simulink model "OpenLoopBraking"  (R2026b)
undefined symbols (not defined in the file): CtrlBcuTrlrBrkGain
settings Model: Creator=The MathWorks, Inc.  LastModifiedBy=The MathWorks, Inc.

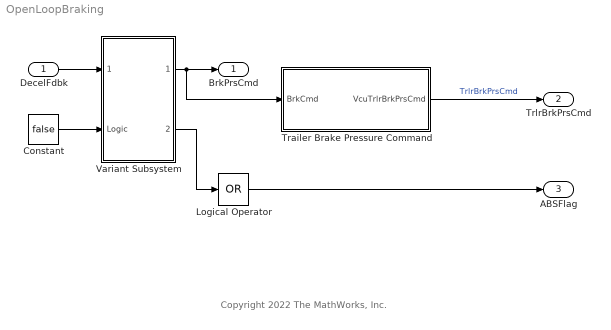
== system OpenLoopBraking ==
  note: Copyright 2022 The MathWorks, Inc.
  DecelFdbk : Inport  OutDataTypeStr=double  PortDimensions=1
  Constant : Constant  Value=false
  Logical Operator : Logic  Operator=OR  Inputs=1  AllPortsSameDT=off  OutDataTypeStr=boolean
  Trailer Brake Pressure Command : Subsystem
  Variant Subsystem : Subsystem  Variant=on  VariantControlMode=label  LabelModeActiveChoice=TwoAxle
  BrkPrsCmd : Outport  OutDataTypeStr=double  VectorParamsAs1DForOutWhenUnconnected=off
  TrlrBrkPrsCmd : Outport  Port=2  PortDimensions=6  VectorParamsAs1DForOutWhenUnconnected=off
  ABSFlag : Outport  Port=3
  wires:
  Variant Subsystem/2(ABSFlag) -> Logical Operator/1
  Constant/1 -> Variant Subsystem/2(Logic)
  Variant Subsystem/1(BrkCmd) -> Trailer Brake Pressure Command/1(BrkCmd), BrkPrsCmd/1
  DecelFdbk/1 -> Variant Subsystem/1(DecelFdbk)
  Trailer Brake Pressure Command/1(VcuTrlrBrkPrsCmd) -> TrlrBrkPrsCmd/1  "TrlrBrkPrsCmd"
  Logical Operator/1 -> ABSFlag/1

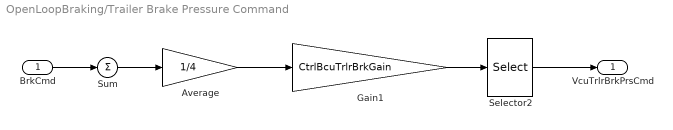
== system OpenLoopBraking/Trailer Brake Pressure Command ==
  BrkCmd : Inport
  Average : Gain  Gain=1/4
  Gain1 : Gain  Gain=CtrlBcuTrlrBrkGain
  Selector2 : Selector  InputPortWidth=1  IndexOptions=Index vector (dialog)  Indices=[1 1 1 1 1 1]  OutputSizes=1  RuntimeRangeChecks=off
  Sum : Sum  Inputs=+
  VcuTrlrBrkPrsCmd : Outport
  wires:
  Gain1/1 -> Selector2/1
  Average/1 -> Gain1/1
  BrkCmd/1 -> Sum/1
  Sum/1 -> Average/1
  Selector2/1 -> VcuTrlrBrkPrsCmd/1

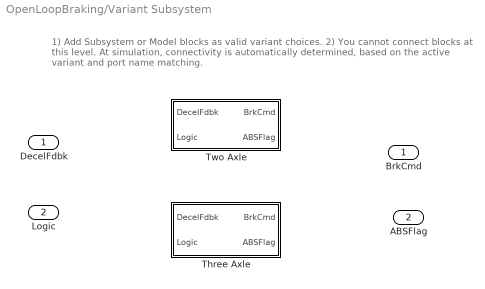
== system OpenLoopBraking/Variant Subsystem ==
  note: 1) Add Subsystem or Model blocks as valid variant choices.
      | 2) You cannot connect blocks at this level. At simulation, connectivity is automatically
      | determined, based on the active variant and port name matching.
  DecelFdbk : Inport
  Logic : Inport  Port=2
  Three Axle : Subsystem  VariantControl=ThreeAxle
  Two Axle : Subsystem  VariantControl=TwoAxle
  BrkCmd : Outport
  ABSFlag : Outport  Port=2

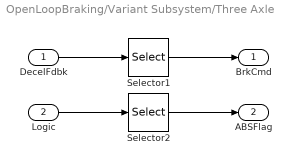
== system OpenLoopBraking/Variant Subsystem/Three Axle ==
  DecelFdbk : Inport
  Logic : Inport  Port=2
  Selector1 : Selector  InputPortWidth=1  IndexOptions=Index vector (dialog)  Indices=[1 1 1 1 1 1]  OutputSizes=1  RuntimeRangeChecks=off
  Selector2 : Selector  InputPortWidth=1  IndexOptions=Index vector (dialog)  Indices=[1 1 1 1 1 1]  OutputSizes=1  RuntimeRangeChecks=off
  BrkCmd : Outport
  ABSFlag : Outport  Port=2
  wires:
  Selector1/1 -> BrkCmd/1
  DecelFdbk/1 -> Selector1/1
  Selector2/1 -> ABSFlag/1
  Logic/1 -> Selector2/1

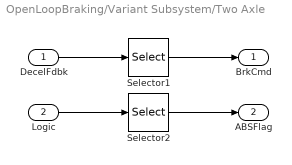
== system OpenLoopBraking/Variant Subsystem/Two Axle ==
  DecelFdbk : Inport
  Logic : Inport  Port=2
  Selector1 : Selector  InputPortWidth=1  IndexOptions=Index vector (dialog)  Indices=[1 1 1 1]  OutputSizes=1  RuntimeRangeChecks=off
  Selector2 : Selector  InputPortWidth=1  IndexOptions=Index vector (dialog)  Indices=[1 1 1 1]  OutputSizes=1  RuntimeRangeChecks=off
  BrkCmd : Outport
  ABSFlag : Outport  Port=2
  wires:
  DecelFdbk/1 -> Selector1/1
  Selector1/1 -> BrkCmd/1
  Logic/1 -> Selector2/1
  Selector2/1 -> ABSFlag/1
